simulink model "Cruise_Control"  (R2019b)
settings: Solver=VariableStepAuto  StartTime=0.0  StopTime=10.0  RelTol=1e-3
values from neighbouring files (symbols this model uses):
  b = 50.0    [Var.sldd]
  m = 1000.0    [Var.sldd]
settings Model: DataDictionary=Var.sldd  Creator=ip  LastModifiedBy=ip
settings DataIOCC: SaveOutput=off  SaveTime=off

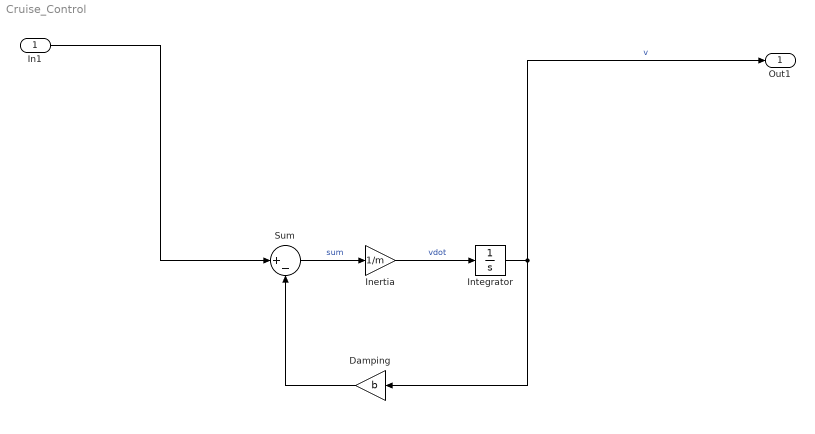
== system Cruise_Control ==
  In1 : Inport  OutDataTypeStr=double  PortDimensions=1  SampleTime=0
  Damping : Gain  Gain=b
  Inertia : Gain  Gain=1/m
  Integrator : Integrator
  Sum : Sum  Inputs=|+-
  Out1 : Outport  OutDataTypeStr=double  PortDimensions=1  SampleTime=0
  wires:
  In1/1 -> Sum/1
  Damping/1 -> Sum/2
  Integrator/1 -> Damping/1, Out1/1  "v"
  Inertia/1 -> Integrator/1  "vdot"
  Sum/1 -> Inertia/1  "sum"
